simulink model "floating_neutral"  (R2014a)
settings: Solver=ode23tb  StartTime=0.0  StopTime=0.1  FixedStep=Ts  MaxStep=1e-3  RelTol=1e-4
PreLoadFcn:
  | Ts=2.5e-5;
InitFcn:
  | Ts=2.5e-5;
libraries: powerlib x9
settings Model: Creator=gdudgeon  LastModifiedBy=cosorio
settings DataIOCC: SignalLoggingSaveFormat=ModelDataLogs
settings OptimizationCC: ExpressionDepthLimit=2147483647  InitFltsAndDblsToZero=on
settings DebuggingCC: SaveWithParameterizedLinksMsg=none  UnderspecifiedInitializationDetection=Classic  SignalResolutionControl=TryResolveAllWithWarning  MultiTaskDSMMsg=warning  MultiTaskCondExecSysMsg=none  FcnCallInpInsideContextMsg=UseLocalSettings  StateNameClashWarn=warning
settings RTWCC: IncludeERTFirstTime=on
settings GRTTargetCC: TargetFcnLib=ansi_tfl_tmw.mat  CombineOutputUpdateFcns=off  GRTInterface=on

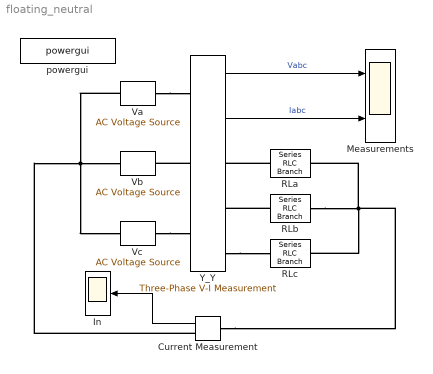
== system floating_neutral ==
  Current Measurement : powerlib/Measurements/Current Measurement  PhasorSimulation=off  OutputType=Complex  PSBequivalent=0
  In : Scope
      settings: YMin=-100  YMax=100
  Measurements : Scope  NumInputPorts=2
      settings: YMin=-200~-100  YMax=200~100
  RLa : powerlib/Elements/Series RLC Branch  LConnTagsString=__new0  RConnTagsString=__new0  BranchType=RL  Resistance=1  Inductance=1e-3  SetiL0=off  InitialCurrent=0  Capacitance=1e-6  Setx0=off  InitialVoltage=0  Measurements=None
  RLb : powerlib/Elements/Series RLC Branch  LConnTagsString=__new0  RConnTagsString=__new0  BranchType=RL  Resistance=1  Inductance=1e-3  SetiL0=off  InitialCurrent=0  Capacitance=1e-6  Setx0=off  InitialVoltage=0  Measurements=None
  RLc : powerlib/Elements/Series RLC Branch  LConnTagsString=__new0  RConnTagsString=__new0  BranchType=RL  Resistance=1  Inductance=1e-3  SetiL0=off  InitialCurrent=0  Capacitance=1e-6  Setx0=off  InitialVoltage=0  Measurements=None
  Va : powerlib/Electrical Sources/AC Voltage Source  Amplitude=100*sqrt(2)/sqrt(3)  Phase=0  Frequency=60  SampleTime=0  Measurements=None
  Vb : powerlib/Electrical Sources/AC Voltage Source  Amplitude=100*sqrt(2)/sqrt(3)  Phase=-120  Frequency=60  SampleTime=0  Measurements=None
  Vc : powerlib/Electrical Sources/AC Voltage Source  Amplitude=100*sqrt(2)/sqrt(3)  Phase=120  Frequency=60  SampleTime=0  Measurements=None
  Y_Y : powerlib/Measurements/Three-Phase V-I Measurement  VoltageMeasurement=phase-to-phase  SetLabelV=off  LabelV=Vabc  Vpu=off  VpuLL=off  CurrentMeasurement=yes  SetLabelI=off  LabelI=Iabc  Ipu=off  Pbase=100e6  Vbase=500e3  OutputType=Complex  PhasorSimulation=off  PSBequivalent=0
  powergui : powerlib/powergui  Priority=2  SimulationMode=Continuous  SolverType=Tustin  SampleTime=Ts  frequency=60  SPID=off  DisableSnubberDevices=off  DisableRonSwitches=off  DisableVfSwitches=off  SwTol=0  Interpol=off  DisplayEquations=off  Ts=0  methode=off  frequencyindice=60  Pbase=100e6  ErrMax=1e-4  Iterations=50  UnitsV=kV  UnitsW=MW  FunctionMessages=off  echomessages=off  HookPort=off  EnableUseOfTLC=off  x0status=blocks  RestoreLinks=warning  ResistiveCurrentMeasurement=off  Frange=[0:2:500]  Ylog=off  Xlog=on  ShowGrid=off  save=off  variable=ZData  structure=Iabc2  ZoomFFT=on  StartTime=4  cycles=1  DisplayStyle=1  fundamental=60  FreqAxis=on  MaxFrequency=2000  frequencyindicesteady=1  RmsSteady=1  display=off
  wires:
  Y_Y/1 -> Measurements/1  "Vabc"
  Y_Y/2 -> Measurements/2  "Iabc"
  Current Measurement/1 -> In/1
  connections:
  RLa/LConn1 -- Y_Y/RConn1
  Y_Y/RConn3 -- RLc/LConn1
  RLb/LConn1 -- Y_Y/RConn2
  Y_Y/LConn2 -- Vb/RConn1
  Va/RConn1 -- Y_Y/LConn1
  Vc/RConn1 -- Y_Y/LConn3
  Va/LConn1 -- Current Measurement/RConn1 -- Vc/LConn1 -- Vb/LConn1
  RLc/RConn1 -- Current Measurement/LConn1 -- RLb/RConn1 -- RLa/RConn1
